simulink model "Safonovo_simplified_inverter"  (R2021b)
settings: Solver=ode23tb  StartTime=0.0  StopTime=30  MaxStep=1e-6  RelTol=5e-4  EnableMultiTasking=on
libraries: spsControlledVoltageSourceLib x3, spsMeanLib x1, spsPermanentMagnetSynchronousMachineLib x1, spspowerguiLib x1
settings Model: Creator=Алексей  LastModifiedBy=alexey
settings SolverCC: ZeroCrossControl=DisableAll  ZeroCrossAlgorithm=Adaptive  AlgebraicLoopSolver=TrustRegion
settings DataIOCC: SaveFormat=Array  SaveOutput=off  DSMLogging=off  SaveTime=off  ReturnWorkspaceOutputs=off
settings OptimizationCC: LifeSpan=inf
settings DebuggingCC: UnderspecifiedInitializationDetection=Classic  MergeDetectMultiDrivingBlocksExec=none  SolverPrmCheckMsg=warning  AllowSymbolicDim=off  SFUnexpectedBacktrackingDiag=warning  SFNoUnconditionalDefaultTransitionDiag=warning  SFExecutionAtInitializationDiag=none  SFMachineParentedDataDiag=warning  ArithmeticOperatorsInVariantConditions=warning
settings HardwareCC: ProdBitPerPointer=32  ProdBitPerSizeT=32  ProdBitPerPtrDiffT=32  ProdLargestAtomicFloat=None  ProdIntDivRoundTo=Undefined  ProdEndianess=Unspecified  ProdWordSize=32  ProdHWDeviceType=32-bit Generic
settings ModelReferenceCC: PropagateSignalLabelsOutOfModel=off
settings SFSimCC: SimUseLocalCustomCode=off  CustomCodeUndefinedFunction=UseInterfaceOnly
settings RTWCC: RTWUseLocalCustomCode=off
settings CodeAppCC: StateflowObjectComments=on
settings GRTTargetCC: TargetLangStandard=C89/C90 (ANSI)
settings ConfigComp: CovMetricSettings=dw  CovSaveCumulativeToWorkspaceVar=on  CovSaveSingleToWorkspaceVar=on  CovExternalEMLEnable=off  CovSFcnEnable=off
settings SimscapeCC: SimscapeNormalizeSystem=off

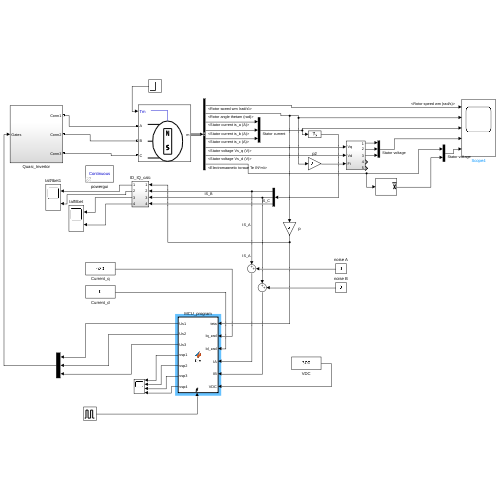
[thumbnail: Simulink's stored preview of the top-level diagram]
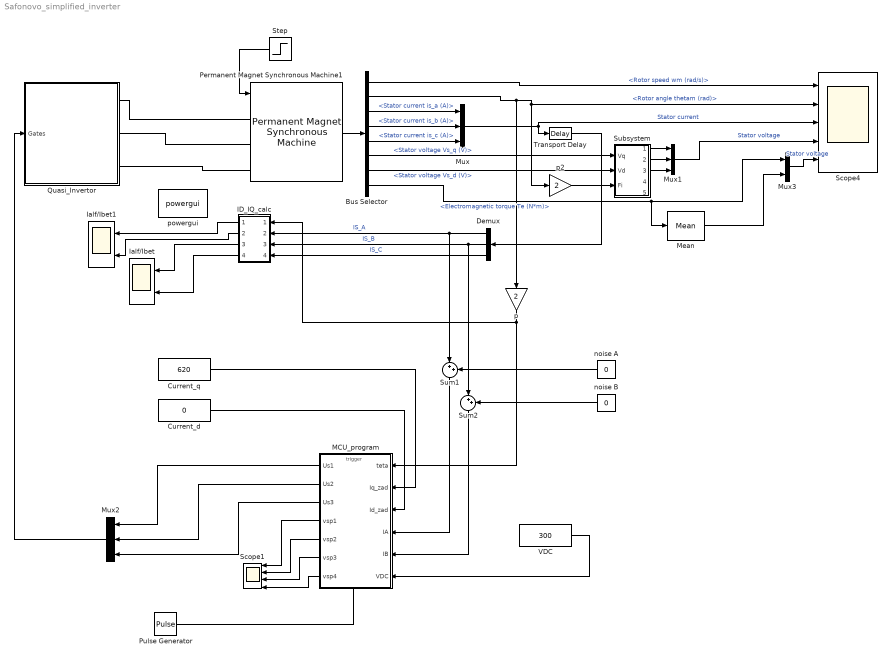
== system Safonovo_simplified_inverter ==
  Bus Selector : BusSelector  OutputSignals=Rotor speed wm (rad/s),Rotor angle thetam (rad),Stator current is_a (A),Stator current is_b (A),Stator current is_c (A),Stator voltage Vs_q (V),Stator voltage Vs_d (V),Electromagnetic torque Te (N*m)
  Current_d : Constant  Value=0
  Current_q : Constant  Value=620
  Demux : Demux  Outputs=3
  ID_IQ_calc : Subsystem
  Ialf/Ibet : Scope  NumInputPorts=2
  Ialf/Ibet1 : Scope  NumInputPorts=2
  MCU_program : MATLAB Function  TreatAsAtomicUnit=on
  Mean : spsMeanLib/Mean  Freq=1000  Vinit=0  Ts=0
  Mux : Mux  Inputs=3
  Mux1 : Mux  Inputs=3
  Mux2 : Mux  Inputs=3
  Mux3 : Mux  Inputs=2
  Permanent Magnet Synchronous Machine1 : spsPermanentMagnetSynchronousMachineLib/Permanent Magnet Synchronous Machine  NbPhases=3  FluxDistribution=Sinusoidal  RotorType=Round  MechanicalLoad=Torque Tm  PresetModel=No  ShowDetailedParameters=on  MeasurementBus=off  Resistance=0.00285  Inductance=8.5e-3  dqInductances=[0.37e-3, 1.075e-3]  La=68.03e-6  MachineConstant=Flux linkage established by magnets (V.s)  Flux=0.0549  VoltageCst=19.9155  TorqueCst=0.1647  Flat=120  Mechanical=[2e104 3e-03 2 0]  PolePairs=1  InitialConditions=[100,0, 0,0]  InitialConditions5ph=[0 0 0 0 0 0]  RefAngle=Aligned with phase A axis (original Park)  IterativeDiscreteModel=Trapezoidal non iterative  TsBlock=-1  TsPowergui=0
  Pulse Generator : DiscretePulseGenerator  PulseType=Time based  Period=50e-6  PulseWidth=10
  Quasi_Invertor : Subsystem
  Scope1 : Scope  NumInputPorts=4
  Scope4 : Scope  NumInputPorts=5
  Step : Step  Time=28  Before=0.02  After=0.07  SampleTime=0
  Subsystem : Subsystem
  Sum1 : Sum  Inputs=|++
  Sum2 : Sum  Inputs=|++
  Transport Delay : TransportDelay  DelayTime=5e-6
  VDC : Constant  Value=300
  noise A : Constant  Value=0
  noise B : Constant  Value=0
  p : Gain  Gain=2
  p2 : Gain  Gain=2
  powergui : spspowerguiLib/powergui  Priority=1  SimulationMode=Continuous  SampleTime=50e-6  frequency=60  Iterations=50  frequencyindice=0  Pbase=100e6  ErrMax=1e-4  UnitsV=kV  UnitsW=MW  buscounter=0  FunctionMessages=off  echomessages=off  EnableUseOfTLC=off  CurrentSourceSwitches=on  DisableSnubberDevices=off  DisableRonSwitches=off  DisableVfSwitches=off  DisplayEquations=off  AutomaticDiscreteSolvers=off  SolverType=Tustin  Interpol=off  ExternalGateDelay=off  methode=off  Ts=0  x0status=blocks  SPID=off  SwTol=0  HookPort=off  NonlinearTolerance=1e-4  nMaxIteration=100  ContinueOnMaxIteration=off  RestoreLinks=warning  ResistiveCurrentMeasurement=off  Frange=[0:2:500]  Ylog=off  Xlog=on  ShowGrid=off  save=off  variable=ZData  structure=SD2  ZoomFFT=on  StartTime=0.7  cycles=10  DisplayStyle=4  fundamental=382  FreqAxis=off  MaxFrequency=50000  frequencyindicesteady=1  RmsSteady=1  display=off
  wires:
  Demux/1 -> ID_IQ_calc/2(In2), Sum1/1  "IS_A"
  Demux/2 -> ID_IQ_calc/3(In3), Sum2/1  "IS_B"
  Permanent Magnet Synchronous Machine1/1 -> Bus Selector/1
  Bus Selector/3 -> Mux/1  "<Stator current is_a (A)>"
  Bus Selector/4 -> Mux/2  "<Stator current is_b (A)>"
  Bus Selector/5 -> Mux/3  "<Stator current is_c (A)>"
  Bus Selector/6 -> Subsystem/1(Vq)  "<Stator voltage Vs_q (V)>"
  Bus Selector/7 -> Subsystem/2(Vd)  "<Stator voltage Vs_d (V)>"
  Subsystem/2(Out2) -> Mux1/2
  Subsystem/3(Out3) -> Mux1/3
  Subsystem/1(Out1) -> Mux1/1
  Mux/1 -> Scope4/3, Transport Delay/1  "Stator current"
  Mux1/1 -> Scope4/4  "Stator voltage"
  Bus Selector/8 -> Mean/1, Mux3/1  "<Electromagnetic torque Te (N*m)>"
  Demux/3 -> ID_IQ_calc/4(In4)  "IS_C"
  Step/1 -> Permanent Magnet Synchronous Machine1/1
  MCU_program/1(Us1) -> Mux2/1
  MCU_program/2(Us2) -> Mux2/2
  MCU_program/3(Us3) -> Mux2/3
  MCU_program/5(vsp2) -> Scope1/2
  MCU_program/6(vsp3) -> Scope1/3
  MCU_program/4(vsp1) -> Scope1/1
  Sum1/1 -> MCU_program/4(IA)
  Sum2/1 -> MCU_program/5(IB)
  Bus Selector/1 -> Scope4/1  "<Rotor speed wm (rad/s)>"
  Bus Selector/2 -> Scope4/2, p2/1, p/1  "<Rotor angle thetam (rad)>"
  Pulse Generator/1 -> MCU_program/Trigger
  Transport Delay/1 -> Demux/1
  noise A/1 -> Sum1/2
  noise B/1 -> Sum2/2
  MCU_program/7(vsp4) -> Scope1/4
  ID_IQ_calc/3(Out3) -> Ialf/Ibet/1
  ID_IQ_calc/4(Out4) -> Ialf/Ibet/2
  p/1 -> MCU_program/1(teta), ID_IQ_calc/1(In1)
  p2/1 -> Subsystem/3(Fi)
  Mux2/1 -> Quasi_Invertor/1(Gates)
  Current_q/1 -> MCU_program/2(Iq_zad)
  Current_d/1 -> MCU_program/3(Id_zad)
  VDC/1 -> MCU_program/6(VDC)
  ID_IQ_calc/1(Out1) -> Ialf/Ibet1/1
  ID_IQ_calc/2(Out2) -> Ialf/Ibet1/2
  Mux3/1 -> Scope4/5  "Stator voltage"
  Mean/1 -> Mux3/2
  connections:
  Permanent Magnet Synchronous Machine1/LConn1 -- Quasi_Invertor/RConn1
  Quasi_Invertor/RConn3 -- Permanent Magnet Synchronous Machine1/LConn3
  Permanent Magnet Synchronous Machine1/LConn2 -- Quasi_Invertor/RConn2

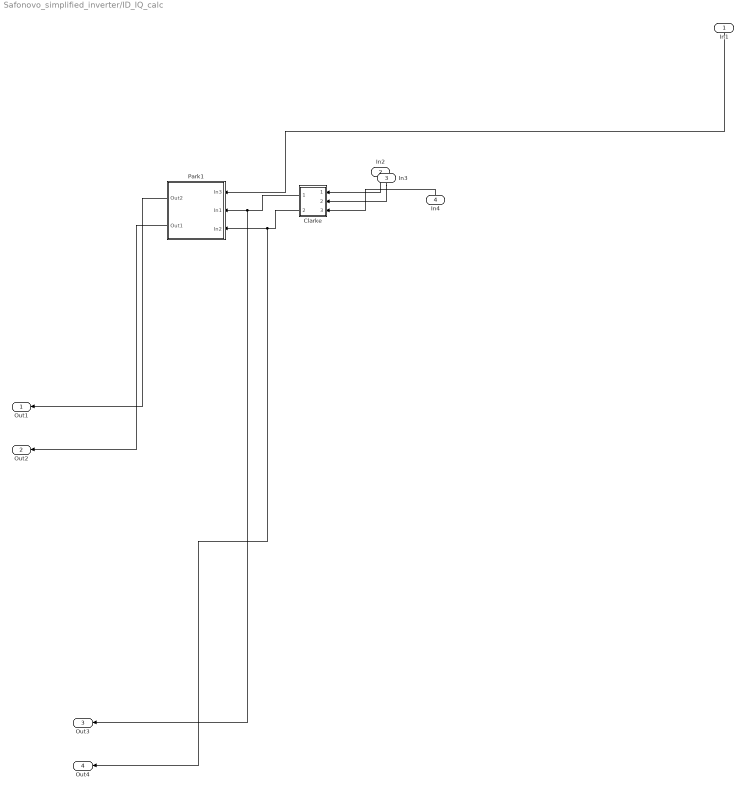
== system Safonovo_simplified_inverter/ID_IQ_calc ==
  In1 : Inport
  In2 : Inport  Port=2
  In3 : Inport  Port=3
  In4 : Inport  Port=4
  Clarke : Subsystem
  Park1 : Subsystem
  Out1 : Outport  VectorParamsAs1DForOutWhenUnconnected=off
  Out2 : Outport  Port=2  VectorParamsAs1DForOutWhenUnconnected=off
  Out3 : Outport  Port=3  VectorParamsAs1DForOutWhenUnconnected=off
  Out4 : Outport  Port=4  VectorParamsAs1DForOutWhenUnconnected=off
  wires:
  Park1/2(Out1) -> Out2/1
  Park1/1(Out2) -> Out1/1
  In1/1 -> Park1/1(In3)
  In4/1 -> Clarke/3(In3)
  In2/1 -> Clarke/1(In1)
  In3/1 -> Clarke/2(In2)
  Clarke/2(Out1) -> Out4/1, Park1/3(In2)
  Clarke/1(Out2) -> Out3/1, Park1/2(In1)

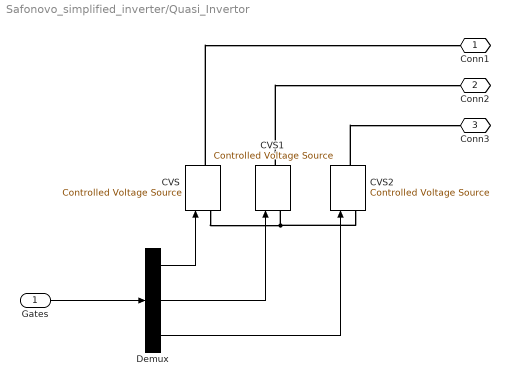
== system Safonovo_simplified_inverter/Quasi_Invertor ==
  Gates : Inport
  CVS : spsControlledVoltageSourceLib/Controlled Voltage Source  Initialize=on  Source_Type=AC  Amplitude=0  Phase=0  Frequency=0  Measurements=None
  CVS1 : spsControlledVoltageSourceLib/Controlled Voltage Source  Initialize=on  Source_Type=AC  Amplitude=0  Phase=0  Frequency=0  Measurements=None
  CVS2 : spsControlledVoltageSourceLib/Controlled Voltage Source  Initialize=on  Source_Type=AC  Amplitude=0  Phase=0  Frequency=0  Measurements=None
  Demux : Demux  Outputs=3
  Conn1 : PMIOPort  Side=Right
  Conn2 : PMIOPort  Port=2  Side=Right
  Conn3 : PMIOPort  Port=3  Side=Right
  wires:
  Demux/1 -> CVS/1
  Demux/2 -> CVS1/1
  Demux/3 -> CVS2/1
  Gates/1 -> Demux/1
  connections:
  CVS1/RConn1 -- Conn2/RConn1
  CVS2/RConn1 -- Conn3/RConn1
  CVS/RConn1 -- Conn1/RConn1
  CVS/LConn1 -- CVS2/LConn1 -- CVS1/LConn1

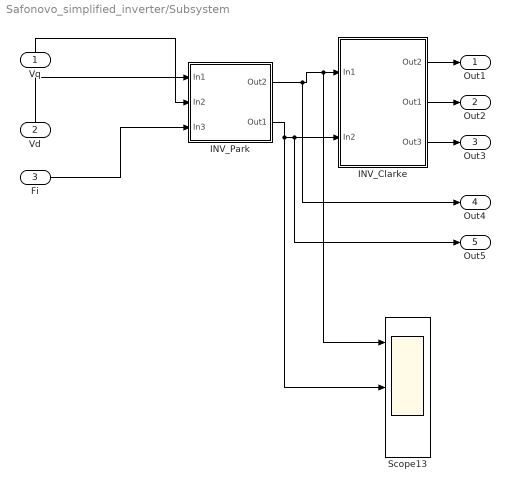
== system Safonovo_simplified_inverter/Subsystem ==
  Vq : Inport
  Vd : Inport  Port=2
  Fi : Inport  Port=3
  INV_Clarke : Subsystem
  INV_Park : Subsystem
  Scope13 : Scope  NumInputPorts=3
  Out1 : Outport  VectorParamsAs1DForOutWhenUnconnected=off
  Out2 : Outport  Port=2  VectorParamsAs1DForOutWhenUnconnected=off
  Out3 : Outport  Port=3  VectorParamsAs1DForOutWhenUnconnected=off
  Out4 : Outport  Port=4  VectorParamsAs1DForOutWhenUnconnected=off
  Out5 : Outport  Port=5  VectorParamsAs1DForOutWhenUnconnected=off
  wires:
  INV_Clarke/2(Out1) -> Out2/1
  INV_Park/1(Out2) -> Out4/1, Scope13/1, INV_Clarke/1(In1)
  INV_Clarke/1(Out2) -> Out1/1
  INV_Park/2(Out1) -> Scope13/2, Out5/1, INV_Clarke/2(In2)
  INV_Clarke/3(Out3) -> Out3/1
  Fi/1 -> INV_Park/3(In3)
  Vd/1 -> INV_Park/1(In1)
  Vq/1 -> INV_Park/2(In2)

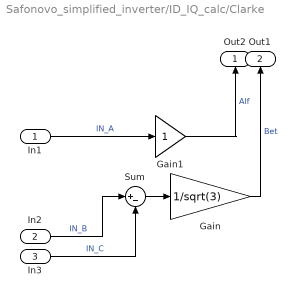
== system Safonovo_simplified_inverter/ID_IQ_calc/Clarke ==
  In1 : Inport
  In2 : Inport  Port=2
  In3 : Inport  Port=3
  Gain : Gain  Gain=1/sqrt(3)
  Gain1 : Gain
  Sum : Sum  Inputs=|+-
  Out2 : Outport  VectorParamsAs1DForOutWhenUnconnected=off
  Out1 : Outport  Port=2  VectorParamsAs1DForOutWhenUnconnected=off
  wires:
  Gain/1 -> Out1/1  "Bet"
  In2/1 -> Sum/1  "IN_B"
  In1/1 -> Gain1/1  "IN_A"
  In3/1 -> Sum/2  "IN_C"
  Sum/1 -> Gain/1
  Gain1/1 -> Out2/1  "Alf"

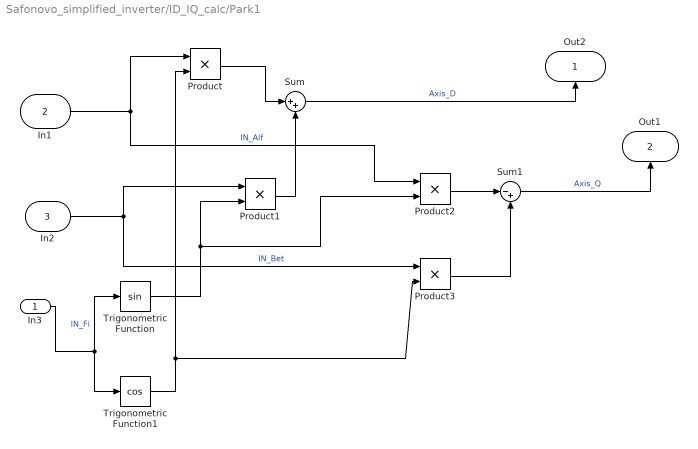
== system Safonovo_simplified_inverter/ID_IQ_calc/Park1 ==
  In3 : Inport
  In1 : Inport  Port=2
  In2 : Inport  Port=3
  Product{,1..3} (4 alike) : Product
  Sum : Sum  Inputs=|++
  Sum1 : Sum  Inputs=|-+
  Trigonometric Function : Trigonometry
  Trigonometric Function1 : Trigonometry  Operator=cos
  Out2 : Outport  VectorParamsAs1DForOutWhenUnconnected=off
  Out1 : Outport  Port=2  VectorParamsAs1DForOutWhenUnconnected=off
  wires:
  Sum1/1 -> Out1/1  "Axis_Q"
  In2/1 -> Product1/1, Product3/1  "IN_Bet"
  In1/1 -> Product2/1, Product/1  "IN_Alf"
  Sum/1 -> Out2/1  "Axis_D"
  In3/1 -> Trigonometric Function1/1, Trigonometric Function/1  "IN_Fi"
  Trigonometric Function1/1 -> Product/2, Product3/2
  Trigonometric Function/1 -> Product2/2, Product1/2
  Product1/1 -> Sum/2
  Product/1 -> Sum/1
  Product2/1 -> Sum1/1
  Product3/1 -> Sum1/2

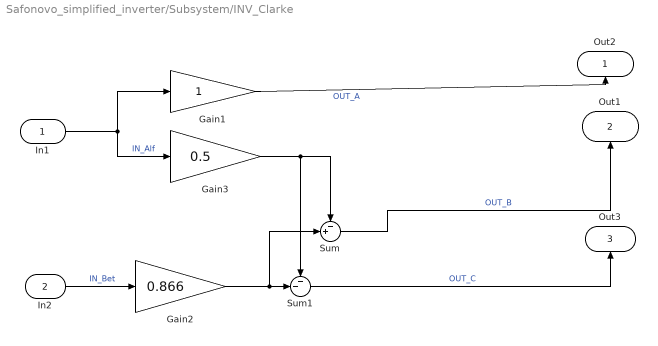
== system Safonovo_simplified_inverter/Subsystem/INV_Clarke ==
  In1 : Inport
  In2 : Inport  Port=2
  Gain1 : Gain
  Gain2 : Gain  Gain=0.866
  Gain3 : Gain  Gain=0.5
  Sum : Sum  Inputs=-+|
  Sum1 : Sum  Inputs=--|
  Out2 : Outport  VectorParamsAs1DForOutWhenUnconnected=off
  Out1 : Outport  Port=2  VectorParamsAs1DForOutWhenUnconnected=off
  Out3 : Outport  Port=3  VectorParamsAs1DForOutWhenUnconnected=off
  wires:
  Sum/1 -> Out1/1  "OUT_B"
  In2/1 -> Gain2/1  "IN_Bet"
  In1/1 -> Gain1/1, Gain3/1  "IN_Alf"
  Gain1/1 -> Out2/1  "OUT_A"
  Sum1/1 -> Out3/1  "OUT_C"
  Gain3/1 -> Sum1/1, Sum/1
  Gain2/1 -> Sum/2, Sum1/2

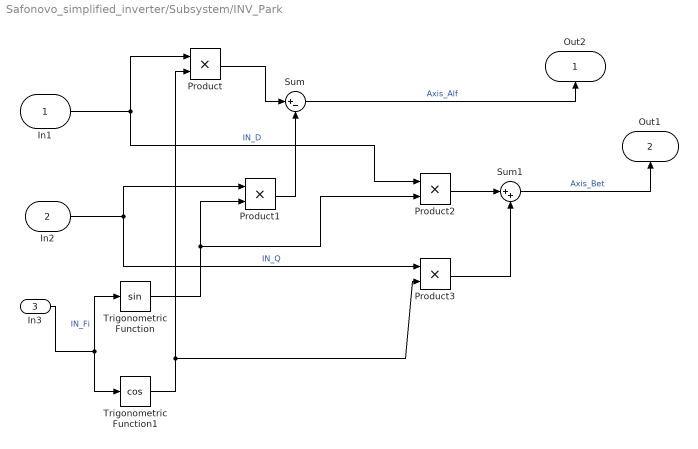
== system Safonovo_simplified_inverter/Subsystem/INV_Park ==
  In1 : Inport
  In2 : Inport  Port=2
  In3 : Inport  Port=3
  Product{,1..3} (4 alike) : Product
  Sum : Sum  Inputs=|+-
  Sum1 : Sum  Inputs=|++
  Trigonometric Function : Trigonometry
  Trigonometric Function1 : Trigonometry  Operator=cos
  Out2 : Outport  VectorParamsAs1DForOutWhenUnconnected=off
  Out1 : Outport  Port=2  VectorParamsAs1DForOutWhenUnconnected=off
  wires:
  Sum1/1 -> Out1/1  "Axis_Bet"
  In2/1 -> Product1/1, Product3/1  "IN_Q"
  In1/1 -> Product2/1, Product/1  "IN_D"
  Sum/1 -> Out2/1  "Axis_Alf"
  In3/1 -> Trigonometric Function1/1, Trigonometric Function/1  "IN_Fi"
  Trigonometric Function1/1 -> Product/2, Product3/2
  Trigonometric Function/1 -> Product2/2, Product1/2
  Product1/1 -> Sum/2
  Product/1 -> Sum/1
  Product2/1 -> Sum1/1
  Product3/1 -> Sum1/2

== matlab function Safonovo_simplified_inverter/MCU_program ==
  data: teta input; Iq_zad input; Id_zad input; IA input; IB input; Us1 output; Us2 output; Us3 output; vsp1 output; vsp2 output; vsp3 output; vsp4 output; VDC input
  events: trigger input RISING_EDGE_EVENT
function [Us1,Us2,Us3,vsp1,vsp2,vsp3,vsp4] = fcn(teta,Iq_zad,Id_zad,IA,IB,VDC)
%время 1/2 ШИМ периода
dt=100e-6;

kuqp=1;
kuqi=25;

kudp=1;
kudi=25;





persistent wint;
if isempty(wint)
    wint=0;
end 
persistent Uqint;
if isempty(Uqint)
    Uqint=0;
end 
persistent Udint;
if isempty(Udint)
    Udint=0;
end 


%Преобразование Кларка
Ialfa=IA;
Ibeta=(2*IB+IA)/sqrt(3);
I_ampl=sqrt(Ialfa^2+Ibeta^2);

%реальные значения токов Id и Iq, полученные через  угол и оси альфа,бета 
Id=Ialfa*cos(teta)+Ibeta*sin(teta);
Iq=Ibeta*cos(teta)-Ialfa*sin(teta); 


%ПИ-регулятор для напряжения по оси Ку
diq=Iq_zad-Iq;
Uqpr=diq*kuqp;
Uqint=Uqint+diq*kuqi*dt;

%ПИ-регулятор для напряжения по оси Дэ
did=Id_zad-Id;
Udpr=did*kudp;
Udint=Udint+did*kudi*dt;

Um=(2/3)*VDC/sqrt(Uqpr^2+Udpr^2);

if(Um<1)
  Uqpr=Uqpr*Um;
  Udpr=Udpr*Um;
end

if((Uqpr+Uqint)>0.85*VDC)
  Uqint=0.85*VDC-Uqpr;
end

if(sqrt((Uqpr+Uqint)^2+(Udpr+Udint)^2)>0.85*VDC)
  Udint=sqrt((0.85*VDC)^2-(Uqpr+Uqint)^2)-Udpr;
end
if(Uqint<0)
  Uqint=0;
end
if(Udint<0)
  Udint=0;
end
  
U_q=Uqpr+Uqint;%+1.5*(L*Idr+psi)*wstart%wrez;                    %15.11 поменял omeg на wrez, интересно, как скажется на точности
U_d=Udpr+Udint;%-1.5*(wstart*Iqr*L);   %wrez      %15.11 поменял omeg на wrez, интересно, как скажется на точности

Ua0=U_d*cos(teta)-U_q*sin(teta);
Ub0=U_d*sin(teta)+U_q*cos(teta);

vrefa=sqrt(Ua0^2+Ub0^2);

if(vrefa>(2/3)*VDC)
  Ua0=Ua0*((2/3)*VDC/vrefa);
  Ub0=Ub0*((2/3)*VDC/vrefa);
end



vsp1=0;
vsp2=0;
vsp3=Id;%wzad-omeg;
vsp4=Iq;



%алгоритм формирования фазных напряжений, КЛАРК


Us1=ceil(Ua0*100)/100;
Us2=sqrt(3)/2*Ub0-0.5*Ua0;
Us2=ceil(Us2*100)/100;
Us3=-0.5*Ua0-sqrt(3)/2*Ub0;
Us3=ceil(Us3*100)/100;




return;
